simulink model "Modelo_Anfis_inverso"  (R2019a)
settings: Solver=VariableStepAuto  StartTime=0.0  StopTime=600  RelTol=1e-3
values from neighbouring files (symbols this model uses):
  Tm = 0.6    [ANFIS_inverso.m]    (also in Codigo_Inverso.m; Codigo_directo.m = 0.2)
libraries: fuzblock x1
settings Model: Creator=Alejoxbg  LastModifiedBy=Jose

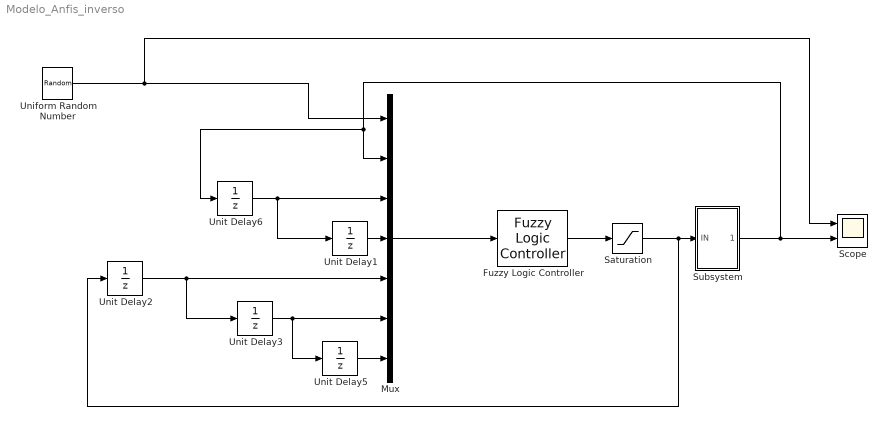
== system Modelo_Anfis_inverso ==
  Fuzzy Logic Controller : fuzblock/Fuzzy Logic  Controller  FIS=fis  OutputSampleNumber=101  DataType=double  FuzzifiedInputs=off  RuleFiringStrengths=off  RuleOutputs=off  AggregatedOutputs=off  SimulateUsing=Interpreted execution  OutOfRangeInputValueMessage=warning  NoRuleFiredMessage=warning  EmptyOutputFuzzySetMessage=warning
  Mux : Mux  Inputs=7
  Saturation : Saturate  UpperLimit=1.7  LowerLimit=0.1
  Scope : Scope  NumInputPorts=2
  Subsystem : Subsystem
  Uniform Random Number : UniformRandomNumber  Minimum=0.2  Seed=11  SampleTime=60
  Unit Delay{1..3,5..6} (5 alike) : UnitDelay  SampleTime=Tm  HasFrameUpgradeWarning=on
  wires:
  Subsystem/1("OUT ") -> Scope/2, Mux/2, Unit Delay6/1
  Saturation/1 -> Unit Delay2/1, Subsystem/1(IN)
  Fuzzy Logic Controller/1 -> Saturation/1
  Mux/1 -> Fuzzy Logic Controller/1
  Unit Delay6/1 -> Unit Delay1/1, Mux/3
  Unit Delay2/1 -> Unit Delay3/1, Mux/5
  Unit Delay1/1 -> Mux/4
  Unit Delay3/1 -> Unit Delay5/1, Mux/6
  Unit Delay5/1 -> Mux/7
  Uniform Random Number/1 -> Mux/1, Scope/1

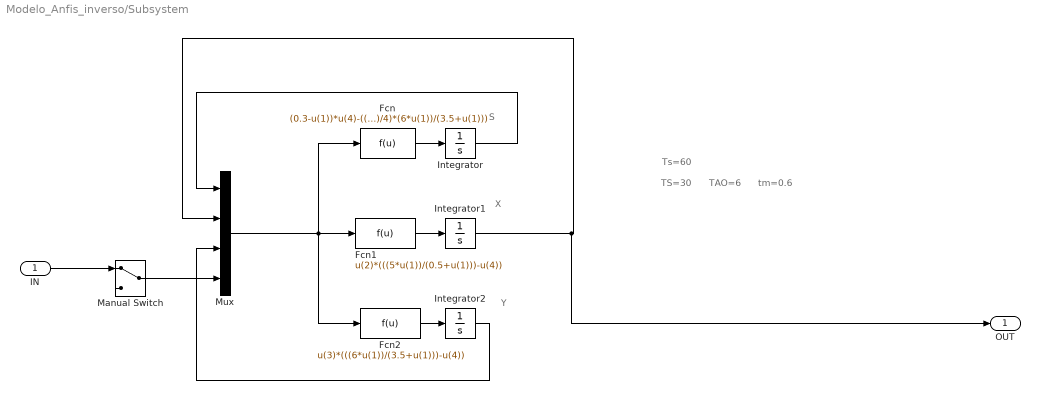
== system Modelo_Anfis_inverso/Subsystem ==
  note: X
  note: Ts=60
  note: S
  note: TAO=6
  note: Y
  note: TS=30
  note: tm=0.6
  IN : Inport
  Fcn : Fcn  Expr=(0.3-u(1))*u(4)-((u(2)/4)*(5*u(1))/(0.5+u(1)))-((u(3)/4)*(6*u(1))/(3.5+u(1)))
  Fcn1 : Fcn  Expr=u(2)*(((5*u(1))/(0.5+u(1)))-u(4))
  Fcn2 : Fcn  Expr=u(3)*(((6*u(1))/(3.5+u(1)))-u(4))
  Integrator : Integrator
  Integrator1 : Integrator  InitialCondition=0.1
  Integrator2 : Integrator
  Manual Switch : ManualSwitch
  Mux : Mux
  "OUT " : Outport
  wires:
  Integrator2/1 -> Mux/3
  Mux/1 -> Fcn/1, Fcn1/1, Fcn2/1
  Fcn2/1 -> Integrator2/1
  Fcn1/1 -> Integrator1/1
  IN/1 -> Manual Switch/1
  Integrator/1 -> Mux/1
  Integrator1/1 -> "OUT "/1, Mux/2
  Manual Switch/1 -> Mux/4
  Fcn/1 -> Integrator/1
